simulink model "ParallelStateMachine"  (R2016a)
settings: Solver=FixedStepAuto  StartTime=0.0  StopTime=inf  RelTol=1e-3
settings Model: ExplicitPartitioning=on  Creator=march  LastModifiedBy=march
settings SolverCC: EnableConcurrentExecution=on  ConcurrentTasks=on
settings GRTTargetCC: GeneratePreprocessorConditionals=Use local settings

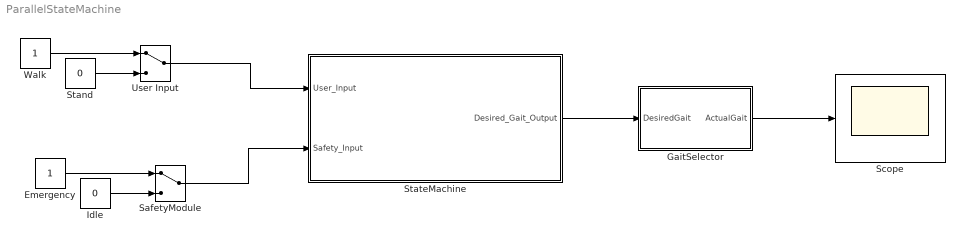
== system ParallelStateMachine ==
  Emergency : Constant
  GaitSelector : Subsystem
  Idle : Constant  Value=0
  SafetyModule : ManualSwitch
  Scope : Scope
  Stand : Constant  Value=0
  StateMachine : Stateflow chart  TreatAsAtomicUnit=on
  User Input : ManualSwitch
  Walk : Constant
  wires:
  SafetyModule/1 -> StateMachine/2(Safety_Input)
  User Input/1 -> StateMachine/1(User_Input)
  Walk/1 -> User Input/1
  Stand/1 -> User Input/2
  Emergency/1 -> SafetyModule/1
  Idle/1 -> SafetyModule/2
  StateMachine/1(Desired_Gait_Output) -> GaitSelector/1(DesiredGait)
  GaitSelector/1(ActualGait) -> Scope/1

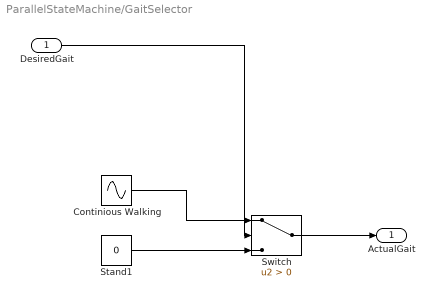
== system ParallelStateMachine/GaitSelector ==
  DesiredGait : Inport
  Continious Walking : Sin  SampleTime=0
  Stand1 : Constant  Value=0
  Switch : Switch  Criteria=u2 > Threshold
  ActualGait : Outport
  wires:
  DesiredGait/1 -> Switch/2
  Switch/1 -> ActualGait/1
  Stand1/1 -> Switch/3
  Continious Walking/1 -> Switch/1

== stateflow chart ParallelStateMachine/StateMachine ==
  state Standing
    entry: Desired_Gait_Output = 0
  state Walking
    entry: Desired_Gait_Output = 1
  (default) -> Standing
  Standing -> Standing [order 2]
  Walking -> Standing [order 1] : [User_Input==0 || Safety_Input==1]
  Standing -> Walking [order 1] : [User_Input>0 && Safety_Input==0]
  Walking -> Walking [order 2]
  data: User_Input input; Safety_Input input; Desired_Gait_Output output
